simulink model "labsetup_cantonisim_distributed"  (R2019a)
settings: Solver=VariableStepAuto  StartTime=0.0  StopTime=100  FixedStep=1  RelTol=1e-3
InitFcn:
  | ini_cantonisim_distributed
values from neighbouring files (symbols this model uses):
  alpha = [0.1853, 0.1187]    [cantoni_LMI_labsetup.m]    (also in distributed_workspace_bak.mat = [0.1853 0.1187])
  kappa = [0.002, 0.003]    [cantoni_LMI_labsetup.m]    (also in distributed_workspace_bak.mat = [0.002 0.003])
  phi = [45, 40]    [cantoni_LMI_labsetup.m]    (also in distributed_workspace_bak.mat = [65 65])
  rho = [1, 1]    [cantoni_LMI_labsetup.m]    (also in distributed_workspace_bak.mat = [1 1])
  S1A = [-967.712947386 4.4408920985e-16 6.10622663544e-16 -1.92592994439e-33 1.7763568394e-15 -967.712947386 -3.5527136788e-15 -1.23259516441e-32 -8.881784197e-16 0 -165.745006005 9.86076131526e-32 ... (16 elements, 4x4)]    [distributed_workspace_bak.mat]
  S1B = [0  0; -1.73472347598e-18  0; -4.85722573274e-17  -2.48689957516e-14; -1.52870689336e-33  6.16297582204e-32]    [distributed_workspace_bak.mat]
  S1C = [0  0  0  0; -0.015989210805  -0.0013940594336  -0.00972898314908  5968537.40601]    [distributed_workspace_bak.mat]
  S1D = [0  0; 6.36918576666e-05  0.470083913441]    [distributed_workspace_bak.mat]
  S2A = [-0.844644033733 -5.20417042793e-18 -1.02348685083e-16 -3.06124483401e-16 0 -0.844644033733 -1.7763568394e-15 -1.52655665886e-15 -4.51028103754e-17 -1.99840144433e-15 -0.841091917384 1.81799020282e-15 ... (16 elements, 4x4)]    [distributed_workspace_bak.mat]
  S2B = [0  0; 0  -2.22044604925e-16; 0  2.6645352591e-15; 0  2.44249065418e-15]    [distributed_workspace_bak.mat]
  S2C = [3.7947076037e-19  1.38777878078e-17  4.16333634234e-17  -0.00457250043278; -0.00323542815991  -0.0125378387304  -0.019389610175  0.0477640488548]    [distributed_workspace_bak.mat]
  S2D = [0  4.16333634234e-17; 0  0.0993341715561]    [distributed_workspace_bak.mat]
  tau = [0.16, 0.1]    [cantoni_LMI_labsetup.m]    (also in distributed_workspace_bak.mat = [0.01 0.05])
  w_n = zeros(1,length(phi_wave))    [cantoni_LMI_labsetup.m]    (also in distributed_workspace_bak.mat = [2.000228049 2.000228049])
  zeta = 0.0151    [cantoni_LMI_labsetup.m]    (also in distributed_workspace_bak.mat)
settings Model: Creator=Jacob  LastModifiedBy=Jacob
settings SolverCC: AlgebraicLoopSolver=LineSearch
settings ModelReferenceCC: ModelReferenceMinAlgLoopOccurrences=on

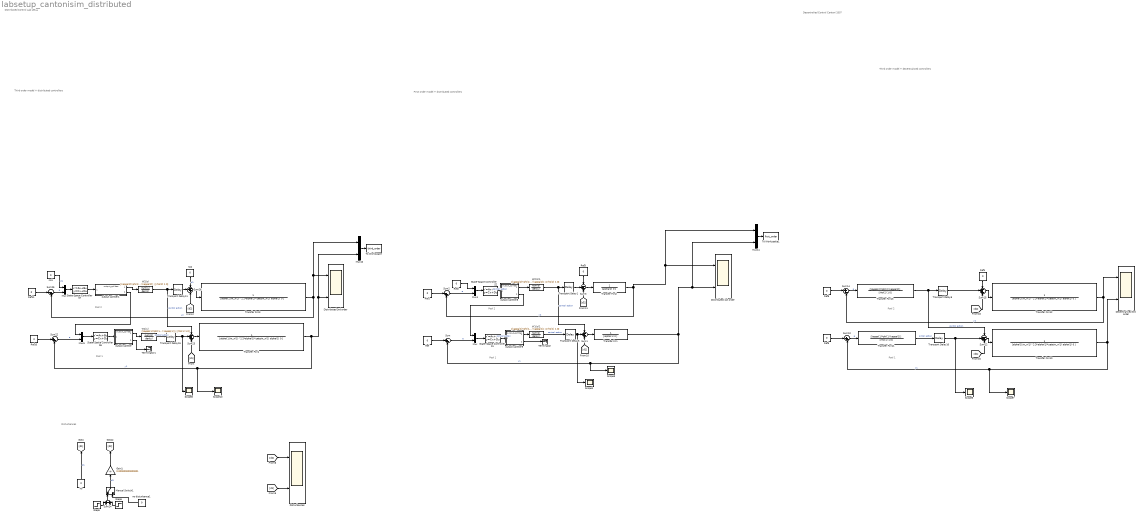
== system labsetup_cantonisim_distributed ==
  note: Disturbances
  note: Decentralied Control Cantoni 2007
  note: Third order model + decentralized controllers
  note: First order model + distributed controllers
  note: Pool 1
  note: Distributed Control Lab Setup
  note: Pool 2
  note: Pool 1
  note: Pool 2
  note: Third order model + distributed controllers
  note: Pool 1
  note: Pool 2
  Decentralized 3rd order : Scope  NumInputPorts=2
  Distributed 1st order : Scope  NumInputPorts=2
  Distributed 3rd order : Scope  NumInputPorts=2
  Disturbances : Scope  NumInputPorts=2
  Gain1 : Gain  Gain=0.000000000000001
  Manual Switch1 : ManualSwitch
  Mux{,1,5..6,10..11} (6 alike) : Mux  Inputs=2
  Ref{,1..6,10..11} (9 alike) : Constant  Value=0
  Scope{1,3,5,7..8,10} (6 alike) : Scope
  State-Space Controller S1 : StateSpace  A=S1A  B=S1B  C=S1C  D=S1D  InitialCondition=0
  State-Space Controller S2 : StateSpace  A=S2A  B=S2B  C=S2C  D=S2D  InitialCondition=0
  State-Space Controller S6 : StateSpace  A=S1A  B=S1B  C=S1C  D=S1D  InitialCondition=0
  State-Space Controller S7 : StateSpace  A=S2A  B=S2B  C=S2C  D=S2D  InitialCondition=0
  Step5 : Step  Time=10  SampleTime=0
  Step6 : Step  Time=20  After=-1  SampleTime=0
  Sum{,10,14,22} (4 alike) : Sum  Inputs=|+-
  Sum{1,3,12,15,23,26} (6 alike) : Sum  Inputs=-++
  Sum2 : Sum  Inputs=|-+
  Sum24 : Sum  Inputs=+|+
  Sum25 : Sum  Inputs=|-+
  Terminator : Terminator
  Terminator1 : Terminator
  To Workspace : ToWorkspace  VariableName=third_order  SaveFormat=Structure With Time  SampleTime=-1
  To Workspace1 : ToWorkspace  VariableName=first_order  SaveFormat=Structure With Time  SampleTime=-1
  Transfer Fcn : TransferFcn  Denominator=[alpha(1) 0 ]
  Transfer Fcn1 : TransferFcn  Denominator=[alpha(1)/w_n(1)^2 2*alpha(1)*zeta/w_n(1) alpha(1) 0 ]
  Transfer Fcn10 : TransferFcn  Denominator=[alpha(1)/w_n(1)^2 2*alpha(1)*zeta/w_n(1) alpha(1) 0 ]
  Transfer Fcn11 : TransferFcn  Numerator=[kappa(1)*phi(1) kappa(1)]  Denominator=[rho(1) 1 0]
  Transfer Fcn12 : TransferFcn  Denominator=[alpha(2)/w_n(2)^2 2*alpha(2)*zeta/w_n(2) alpha(2) 0 ]
  Transfer Fcn13 : TransferFcn  Numerator=[kappa(2)*phi(2) kappa(2)]  Denominator=[rho(2) 1 0]
  Transfer Fcn2 : TransferFcn  Denominator=[alpha(2) 0 ]
  Transfer Fcn3 : TransferFcn  Denominator=[alpha(2)/w_n(2)^2 2*alpha(2)*zeta/w_n(2) alpha(2) 0 ]
  Transport Delay1 : TransportDelay  DelayTime=tau(2)
  Transport Delay10 : TransportDelay  DelayTime=tau(1)
  Transport Delay11 : TransportDelay  DelayTime=tau(2)
  Transport Delay15 : TransportDelay  DelayTime=tau(1)
  Transport Delay5 : TransportDelay  DelayTime=tau(1)
  Transport Delay6 : TransportDelay  DelayTime=tau(2)
  W1(s) : TransferFcn  Numerator=[kappa(1)*phi(1) kappa(1)]  Denominator=[rho(1) 1 0]
  W1(s)1 : TransferFcn  Numerator=[kappa(1)*phi(1) kappa(1)]  Denominator=[rho(1) 1 0]
  W2(s) : TransferFcn  Numerator=[kappa(2)*phi(2) kappa(2)]  Denominator=[rho(2) 1 0]
  W2(s)1 : TransferFcn  Numerator=[kappa(2)*phi(2) kappa(2)]  Denominator=[rho(2) 1 0]
  no : Constant  Value=0
  no disturbance1 : Constant  Value=0
  no1 : Constant  Value=0
  no2 : Constant  Value=0
  output splitter{,1,8..9} (4 alike) : ModelReference  ModelNameDialog=output_splitter  SimulationMode=Normal  ModelReferenceVersion=1.52
  wires:
  W1(s)1/1 -> Transport Delay5/1  "control action"
  Sum/1 -> Mux/2  "e"
  Ref/1 -> Sum/1
  Transport Delay5/1 -> Scope1/1, Sum1/2
  Sum1/1 -> Transfer Fcn/1
  [d1] -> Sum1/3
  Transport Delay1/1 -> Sum3/2
  Transfer Fcn2/1 -> Sum2/2, Mux11/1, Distributed 1st order/1  "y2"
  Sum3/1 -> Transfer Fcn2/1
  W2(s)1/1 -> Sum1/1, Transport Delay1/1  "control action"
  Sum2/1 -> Mux1/2  "e"
  [d2] -> Sum3/3
  Transfer Fcn/1 -> Scope3/1, Sum/2, Mux11/2, Distributed 1st order/2  "y1"
  Ref1/1 -> Sum2/1
  Transport Delay10/1 -> Scope5/1, Sum12/2
  Sum12/1 -> Transfer Fcn10/1
  [d1] -> Sum12/3
  Sum15/1 -> Transfer Fcn12/1
  Sum14/1 -> Transfer Fcn13/1  "e"
  Sum10/1 -> Transfer Fcn11/1  "e"
  Transport Delay6/1 -> Sum15/2
  Transfer Fcn13/1 -> Sum12/1, Transport Delay6/1  "control action"
  Ref6/1 -> Sum14/1
  Transfer Fcn12/1 -> Decentralized 3rd order/1, Sum14/2  "y2"
  [d2] -> Sum15/3
  Transfer Fcn10/1 -> Decentralized 3rd order/2, Scope7/1, Sum10/2  "y1"
  Ref5/1 -> Sum10/1
  Transfer Fcn11/1 -> Transport Delay10/1  "ontrol action"
  Mux/1 -> State-Space Controller S1/1
  Mux1/1 -> State-Space Controller S2/1
  Mux6/1 -> State-Space Controller S7/1
  Mux5/1 -> State-Space Controller S6/1
  [d2] -> Sum26/3
  Transfer Fcn3/1 -> Distributed 3rd order/1, Mux10/1, Sum25/2  "y2"
  Sum26/1 -> Transfer Fcn3/1
  Transport Delay15/1 -> Scope8/1, Sum23/2
  Sum22/1 -> Mux5/2  "e"
  Transport Delay11/1 -> Sum26/2
  Transfer Fcn1/1 -> Scope10/1, Sum22/2, Mux10/2, Distributed 3rd order/2  "y1"
  W1(s)/1 -> Transport Delay15/1  "control action"
  W2(s)/1 -> Sum23/1, Transport Delay11/1  "control action"
  Ref10/1 -> Sum22/1
  Ref11/1 -> Sum25/1
  Sum23/1 -> Transfer Fcn1/1
  Sum25/1 -> Mux6/2  "e"
  [d1] -> Sum23/3
  no disturbance1/1 -> Manual Switch1/2
  Step5/1 -> Sum24/1
  Sum24/1 -> Manual Switch1/1
  Step6/1 -> Sum24/2
  Manual Switch1/1 -> Gain1/1  "d3"
  no/1 -> [d1]  "d1"
  [d1] -> Disturbances/2
  [d2] -> Disturbances/1
  State-Space Controller S6/1 -> output splitter/1
  State-Space Controller S7/1 -> output splitter1/1
  output splitter1/2 -> Mux5/1
  output splitter/1 -> W1(s)/1
  output splitter1/1 -> W2(s)/1
  Gain1/1 -> [d2]
  State-Space Controller S2/1 -> output splitter8/1  "control action"
  output splitter8/1 -> W2(s)1/1
  output splitter8/2 -> Mux/1
  State-Space Controller S1/1 -> output splitter9/1  "control action"
  output splitter9/1 -> W1(s)1/1
  Mux10/1 -> To Workspace/1
  Mux11/1 -> To Workspace1/1
  no1/1 -> Mux6/1  "d1"
  Ref2/1 -> Mux1/1
  no2/1 -> Sum26/1  "d1"
  Ref3/1 -> Sum3/1
  Ref4/1 -> Sum15/1
  output splitter9/2 -> Terminator/1
  output splitter/2 -> Terminator1/1
